simulink model "MecanumPose_18b"  (R2018b)
settings: Solver=VariableStepAuto  StartTime=0.0  StopTime=inf  RelTol=1e-3
InitFcn:
  | mecanum_init
values from neighbouring files (symbols this model uses):
  J = (1/r)*[1 1 a+b ... (first row only)    [mecanum_init.m]
  J3 = (1/r)*[1 1 a+b ... (first row only)    [mecanum_init.m]
libraries: aerolibutil x1, aerolibanimutils x1, robotlib x1
settings Model: Creator=giull  LastModifiedBy=giull
settings DataIOCC: ReturnWorkspaceOutputs=on

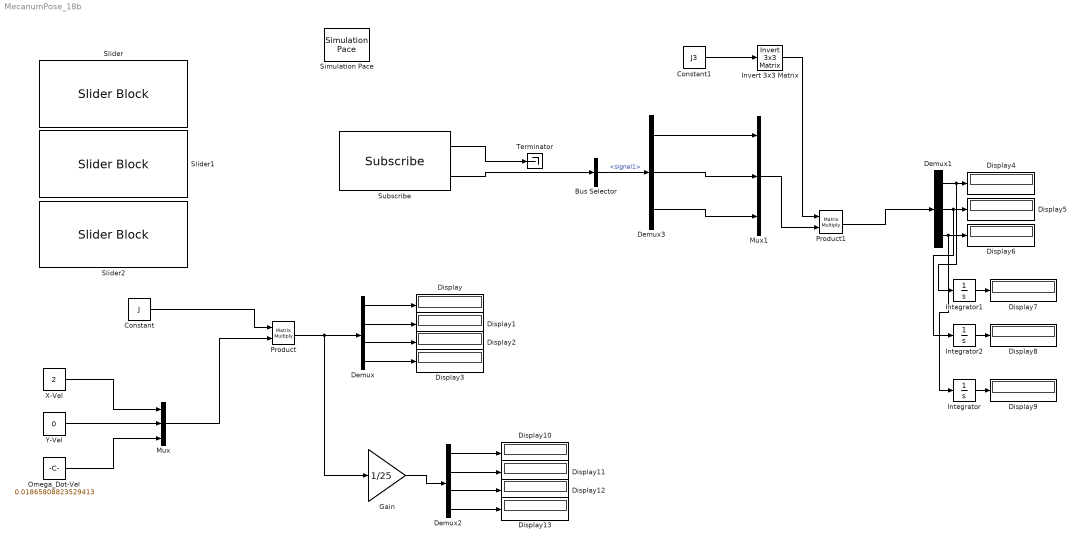
== system MecanumPose_18b ==
  Bus Selector : BusSelector  OutputSignals=signal1
  Constant : Constant  Value=J
  Constant1 : Constant  Value=J3
  Demux : Demux
  Demux1 : Demux  Outputs=3
  Demux2 : Demux
  Demux3 : Demux  Outputs=3
  Display{,1..13} (14 alike) : Display
  Gain : Gain  Gain=1/25
  Integrator : Integrator
  Integrator1 : Integrator
  Integrator2 : Integrator
  Invert 3x3 Matrix : aerolibutil/Invert  3x3 Matrix
  Mux : Mux  Inputs=3
  Mux1 : Mux  Inputs=3
  Omega_Dot-Vel : Constant  Value=0.01865808823529413
  Product : Product  Multiplication=Matrix(*)
  Product1 : Product  Multiplication=Matrix(*)
  Simulation Pace : aerolibanimutils/Simulation Pace  SimulationPace=1  SleepMode=Auto  OutputPaceError=off  SampleTime=1/30
  Slider : SliderBlock  ScaleMin=-2  ScaleMax=2  WebBlockId=13
  Slider1 : SliderBlock  ScaleMin=-2  ScaleMax=2  WebBlockId=15
  Slider2 : SliderBlock  ScaleMin=-0.5  ScaleMax=0.5  WebBlockId=16
  Subscribe : robotlib/Subscribe  topicSource=Specify your own  topic=/CANread  messageType=geometry_msgs/Point  sampleTime=-1  messageQueueLength=1
      settings: SourceProductName=ROS Toolbox
  Terminator : Terminator
  X-Vel : Constant  Value=2
  Y-Vel : Constant  Value=0
  wires:
  Constant/1 -> Product/1
  Y-Vel/1 -> Mux/2
  X-Vel/1 -> Mux/1
  Omega_Dot-Vel/1 -> Mux/3
  Product/1 -> Gain/1, Demux/1
  Mux/1 -> Product/2
  Demux/2 -> Display1/1
  Demux/1 -> Display/1
  Demux/3 -> Display2/1
  Demux/4 -> Display3/1
  Constant1/1 -> Invert 3x3 Matrix/1
  Product1/1 -> Demux1/1
  Demux1/1 -> Integrator1/1, Display4/1
  Demux1/2 -> Integrator2/1, Display5/1
  Demux1/3 -> Integrator/1, Display6/1
  Invert 3x3 Matrix/1 -> Product1/1
  Integrator/1 -> Display9/1
  Integrator2/1 -> Display8/1
  Integrator1/1 -> Display7/1
  Demux2/3 -> Display12/1
  Demux2/2 -> Display11/1
  Demux2/4 -> Display13/1
  Demux2/1 -> Display10/1
  Gain/1 -> Demux2/1
  Mux1/1 -> Product1/2
  Subscribe/2 -> Bus Selector/1
  Subscribe/1 -> Terminator/1
  Bus Selector/1 -> Demux3/1  "<signal1>"
  Demux3/1 -> Mux1/1
  Demux3/2 -> Mux1/2
  Demux3/3 -> Mux1/3
